simulink model "ClimberRobotModel"  (R2020a)
settings: Solver=VariableStepAuto  StartTime=0.0  StopTime=10.0  RelTol=1e-3
settings Model: Creator=danielefontanelli  LastModifiedBy=danielefontanelli

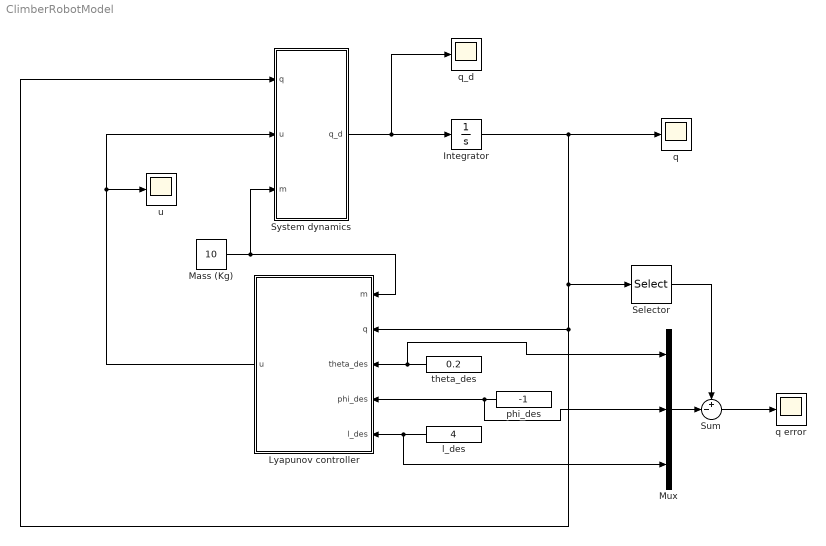
== system ClimberRobotModel ==
  Integrator : Integrator  InitialCondition=rand(6,1)
  Lyapunov controller : MATLAB Function  TreatAsAtomicUnit=on
  Mass (Kg) : Constant  Value=10
  Mux : Mux  Inputs=3
  Selector : Selector  InputPortWidth=6  IndexOptions=Index vector (dialog)  Indices=[1 2 3]  OutputSizes=1
  Sum : Sum  Inputs=+-|
  System dynamics : MATLAB Function  TreatAsAtomicUnit=on
  l_des : Constant  Value=4
  phi_des : Constant  Value=-1
  q : Scope
  q error : Scope
  q_d : Scope
  theta_des : Constant  Value=0.2
  u : Scope
  wires:
  Mass (Kg)/1 -> Lyapunov controller/1(m), System dynamics/3(m)
  System dynamics/1(q_d) -> q_d/1, Integrator/1
  Integrator/1 -> q/1, System dynamics/1(q), Lyapunov controller/2(q), Selector/1
  Lyapunov controller/1(u) -> u/1, System dynamics/2(u)
  theta_des/1 -> Mux/1, Lyapunov controller/3(theta_des)
  phi_des/1 -> Mux/2, Lyapunov controller/4(phi_des)
  l_des/1 -> Mux/3, Lyapunov controller/5(l_des)
  Selector/1 -> Sum/1
  Mux/1 -> Sum/2
  Sum/1 -> q error/1

== matlab function ClimberRobotModel/Lyapunov controller ==
  data: m input; q input; u output; theta_des input; phi_des input; l_des input
function u = fcn(m, q, theta_des, phi_des, l_des)

g = 9.8;   % m/s^2

% Gains
k_theta = 10;
k_phi = 10;
k_l = 10;
k_omega = 1;
k_psi = 1;
k_r = 1;

% State space variables
theta = q(1);
phi = q(2);
l = q(3);
omega = q(4);
psi = q(5);
r = q(6);

% Desired velocities
omega_des = -k_theta*(theta - theta_des);
psi_des = -k_phi*(phi - phi_des);
r_des = -k_l*(l - l_des);

% Value of the nonlinear dynamics
f4 = - 2*omega*r/l + psi^2*sin(theta)*cos(theta) - g/l*sin(theta);
f5 = - 2*psi*r/l - 2*psi*omega*cos(theta)/sin(theta);
f6 = l*(omega^2 + psi^2*sin(theta)^2) + g*cos(theta);

% Control laws
Fn = -m*l*(f4 + k_omega*(omega - omega_des) + k_theta*omega);
Ft = -m*l*sin(theta)*(f5 + k_psi*(psi - psi_des) + k_phi*psi);
Fr = -m*(f6 + k_r*(r - r_des) + k_l*r);

% Controls
u = [Fn, Ft, Fr]';

== matlab function ClimberRobotModel/System dynamics ==
  data: q input; u input; m input; q_d output
function q_d = fcn(q, u, m)

g = 9.8;   % m/s^2

% Inputs
Fn = u(1);
Ft = u(2);
Fr = u(3);

% State space variables
theta = q(1);
phi = q(2);
l = q(3);
omega = q(4);
psi = q(5);
r = q(6);

% Dynamics
theta_p = omega;
phi_p = psi;
l_p = r;
omega_p = - 2*omega*r/l + psi^2*sin(theta)*cos(theta) - g/l*sin(theta) + Fn/(m*l);
psi_p = - 2*psi*r/l - 2*psi*omega*cos(theta)/sin(theta) + Ft/(m*l*sin(theta));
r_p = l*(omega^2 + psi^2*sin(theta)^2) + g*cos(theta) + Fr/m;

% Outputs
q_d = [theta_p, phi_p, l_p, omega_p, psi_p, r_p]';
